simulink model "PTC_EL_PDgJLA_FracPol_20201"  (R2020b)
settings: Solver=VariableStepAuto  StartTime=0.0  StopTime=10.0  RelTol=1e-3
settings Model: Creator=Amir  LastModifiedBy=Amir

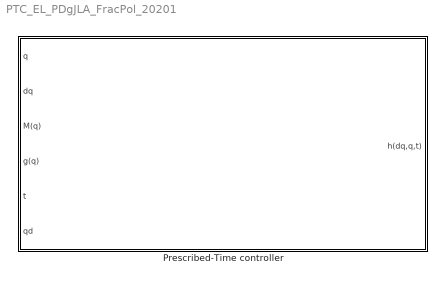
== system PTC_EL_PDgJLA_FracPol_20201 ==
  Prescribed-Time controller : Subsystem  mask(Prescribed-Time Control for Robotics Systems - Version: PTC.EL.PDg-JLA.FracPol.2020-1){n=2, tau=20, P=-0.1*eye(2), D=-1*eye(2), checkBoxA=on, grav_onoff=1, checkBoxB=on, avoid_onoff=1, qmax=[inf;3*pi/180], qmin=[-inf;-3*pi/180], infl=0.5*pi/180, eta=[0;1e-9], a=20, b=1, c=1, epsilon_t=1, epsilon_x=0}
      mask prompts: n "Degrees of Freedom (n):"; tau "Stabilization time (tau):"; P "Proportional (P):"; D "Derivative (D):"; checkBoxA "Gravity compensation"; checkBoxB "Joint limit avoidance"; qmax "Maximum limits (q_max):"; qmin "Minimum limits (q_min):"; infl "Distance limit of influence:"; eta "Joint limit force gain:"
      mask Help:
      | This simulink block obtains a prescribed-time control for Euler-Lagrnage systems of the following form:
      | 
      | M(q)*q+C(dq,q)*dq+g(q)=u+d(t)
      | 
      | where the position of the robot is 'q' and its time derivative is shown by 'dq'. Matrices 'M(q)' and 'C(dq,q)' are the inertia and Coriolis matrices, respectively. Vector 'g(q)' is the gravity force and 'u' stands for the control input. The unmodeled perturbations are refered to by 'd(t)'.
      | 
      | The prescribed-time controller stabilizes the above-mentioned Euler-Lagrange system at 't=tau'.
      | 
      | The parameters of this block are:
      | 
      | 1) n: The degrees of freedom (DOF) of the robot, i.e., the dimension of vector 'q'.
      | 
      | 2) tau: The intended convergence time.
      | 
      | 3) P: The proportional matrix of the infinite-time controller.
      | 
      | 4) D: The derivative matrix of the infinite-time controller.
      | 
      | 5) Gravity compensation checkbox: Infinite-time controller with or whithout gravity compensation.
      | 
      | 6) Joint limit avoidance checkbox: Infinite-time controller with or without joint limit avoidance (use only for revolute joints).
      | 
      | 7) qmax: Maximum limit of the joint angle as a n-dimensional vector.
      | 
      | 8) qmin: Minimum limit of the joint angle as a n-dimensional vector.
      | 
      | 9) Distance limit of influence: Distance limit of the potential field influence; larger values influences the robot even far from the joint limits.
      | 
      | 10) Joint limit force gain: A gain for the joint limit avoidance force.
      | 
      | 11) a: The numinator coefficient for a polynomial mapping function; set an m-dimensional vector to have a mapping function by sum of m polynomial terms.
      | 
      | 12) b: The nominator power for a polynomial mapping function; set an m-dimensional vector to have a mapping function by sum of m polynomial terms.
      | 
      | 13) c: The denominator power for a polynomial mapping function; set an m-dimensional vector to have a mapping function by sum of m polynomial terms.
      | 
      | 14) epsilon_t: For a time-dependent switching, the controller switches to fixed gains at t=tau-epsilon_t.
      | 
      | 15) epsilon_x: For a state-dependent switching, the controller switches to fixed gains when norm(x)<epsilon_x.
      mask Callback checkBoxA:
      | box_A = get_param(gcb, 'checkBoxA');
      | m = Simulink.Mask.get(gcb);
      | 
      | if strcmp(box_A, 'on')
      |     set_param(gcb,'grav_onoff','1')
      | %     grav_onoff=1;
      | else
      |     set_param(gcb,'grav_onoff','0')
      | %     grav_onoff=0;
      | end
      mask Callback checkBoxB:
      | box_B = get_param(gcb, 'checkBoxB');
      | m = Simulink.Mask.get(gcb);
      | m1 = m.getParameter('qmax');
      | m2 = m.getParameter('qmin');
      | m3 = m.getParameter('infl');
      | m4 = m.getParameter('eta');
      | 
      | if strcmp(box_B, 'on')
      |     m1.Enabled = 'on';
      |     m2.Enabled = 'on';
      |     m3.Enabled = 'on';
      |     m4.Enabled = 'on';
      |     set_param(gcb,'avoid_onoff','1')
      | %     avoid_onoff=1;
      | else
      |     m1.Enabled = 'off';
      |     m2.Enabled = 'off';
      |     m3.Enabled = 'off';
      |     m4.Enabled = 'off';
      |     set_param(gcb,'avoid_onoff','0')
      | %     avoid_onoff=0;
      | end
      mask DialogControl DescGroupVar Prompt: Main
      mask DialogControl DescTextVar Prompt: This block obtains a prescribed-time control for robotics system governed by Euler-Lagrange systems.
      mask DialogControl Control5 Prompt: The controller can be set to avoid maximum and minimum limits for revolute joints.
      mask DialogControl Control6 Prompt: The stabilization occurs at 't=tau'. The controller switches to a fixed gain scheme at 't=tau-epsilon_t', or when the norm of state variables reaches a tolerance of 'epsilon_x'.
      mask DialogControl DescTextVar_copy Prompt: This version is based on a Proportional Derivative (PD) controller with/without gravity compensation as the core infinite-time controller. The mapping function is a sum of fractions of polynomials.
      mask DialogControl Container4 Prompt: Parameters
      mask DialogControl ParameterGroupVar Prompt: Basics:
      mask DialogControl ParameterGroupVar_copy_copy Prompt: Joint limits
      mask DialogControl ParameterGroupVar_copy Prompt: Mapping details
      mask DialogControl ParameterGroupVar_copy_copy_copy Prompt: Switching criteria
      mask DialogControl Container6 Prompt: More
      mask DialogControl Control3 Prompt: For updated versions, other versions of prescribed-time control, and more stuff, refer to the following link:
      mask DialogControl Control4 Prompt: https://github.com/a-shakouri
      mask DialogControl Control4 Callback: web https://github.com/a-shakouri
      mask Display:
      | color('red');
      | disp('Joint Limit Avoidance\n Prescribed-Time Control\n for Robotics Systems\n\n Version: PTC.EL.PDg-JLA.FracPol.2020-1')
      | color('blue');
      | port_label('output',1,'controller (u)','texmode','on');
      | port_label('input',1,'position (q)','texmode','on');
      | port_label('input',2,'velocity (dq/dt)','texmode','on');
      | port_label('input',3,'Inertia matrix (M(q))','texmode','on');
      | port_label('input',4,'Gravity (g(q))','texmode','on');
      | port_label('input',5,'Time (t)','texmode','on');
      | port_label('input',6,'Reference position (q_d)','texmode','on');

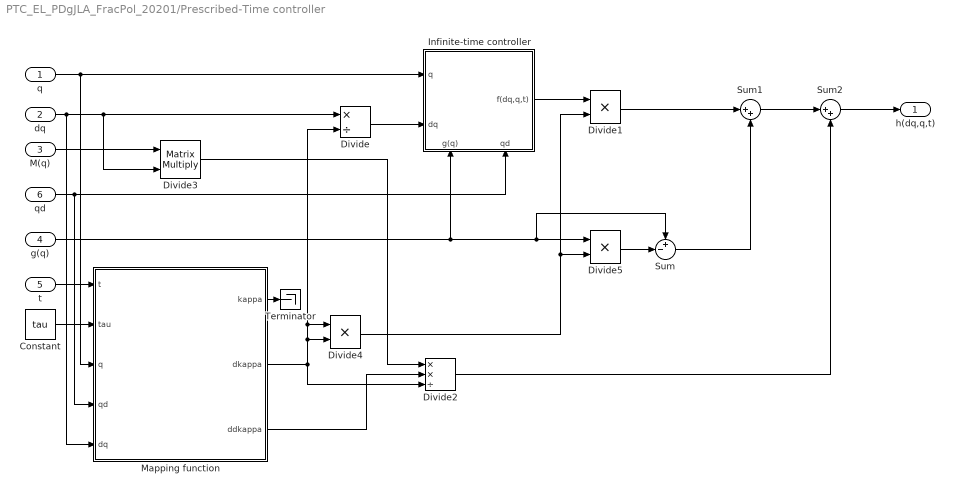
== system PTC_EL_PDgJLA_FracPol_20201/Prescribed-Time controller ==
  q : Inport
  dq : Inport  Port=2
  M(q) : Inport  Port=3
  g(q) : Inport  Port=4
  t : Inport  Port=5
  qd : Inport  Port=6
  Constant : Constant  Value=tau
  Divide : Product  Inputs=*/
  Divide1 : Product  Inputs=**
  Divide2 : Product  Inputs=**/
  Divide3 : Product  Inputs=**  Multiplication=Matrix(*)
  Divide4 : Product  Inputs=**
  Divide5 : Product  Inputs=**
  Infinite-time controller : Subsystem
      settings: PortSchema="{\"entries\":[{\"content\":{\"sides\":[{\"content\":{\"connectorIds\":[\"In1\",\"In2\"]},\"type\":\"ConnectorPlacement.EquallySpacedRectSide\",\"uuid\":\"7fa92645-5ad5-4dcc-b988-cb5fc0cde25c\"},{\"content\":{\"connectorIds\":[\"Out1\"],\"side\":\"RIGHT\"},\"type\":\"ConnectorPlacement.EquallySpacedRectSide\",\"uuid\":\"c20d7c6d-79fc-4692-98a2-c9d8ae7aa432\"},{\"content\":{\"connectorIds\":[],\"side\":\"TOP\"},\"type\":\"ConnectorPlacement.EquallySpacedRectSide\",\"uuid\":\"509ceb5e-78fa-4200-8b36-95fce9268002\"},{\"content\":{\"connectorIds\":[\"In3\",\"In4\"],\"side\":\"BOTTOM\"},\"type\":\"ConnectorPlacement.EquallySpacedRectSide\",\"uuid\":\"0712c4cc-40fb-4aea-b6ca-fbdd2235494d\"},{\"content\":{\"connectorIds\":[],\"side\":\"HIDDEN\"},\"type\":\"ConnectorPlacement.EquallySpacedRectSide\",\"uuid\":\"dedad4c9-c57d-4507-80e4-7406b4950423\"}]},\"type\":\"ConnectorPlacement.EquallySpacedConnector\",\"uuid\":\"14c606af-fbb3-4308-b541-68782b857af4\"}],\"packageUris\":[\"http://schema.mathworks.com/mf0/Connector/R2020b\"],\"version\":\"1.0\"}"
  Mapping function : Subsystem  mask(Polynomial Mapping Function of Class K){a=a, b=b, c=c, Num=0, epsilon_t_copy=epsilon_t, epsilon_x_copy=epsilon_x}
      mask prompts: epsilon_t_copy "epsilon_t:"; epsilon_x_copy "epsilon_x:"
      mask init:
      | Num=length(a);
      mask Help:
      | This simulink block creates the mapping function as well as its first and second derivatives. The mapping functions are of class K such that they go to infinity when the argument approaches t=tau.
      | 
      | The formula of the mapping function (interpreted in LaTeX) is $sum_{i=1}^N(a_i\frac{t^{b_i}}{(\tau-t)^{c_i}})$.
      mask DialogControl DescGroupVar Prompt: Main
      mask DialogControl DescTextVar Prompt: This block obtains the class K mapping function as well as its first and second derivatives for the prescribed-time control of robotics systems. The output limits go to infinity when time approaches 't=tau'. For more details about the following parameters, click on the help button.
      mask DialogControl DescTextVar_copy_copy Prompt: The mapping function ceases updating and returns the latest calculated values after the norm of state variables reaches a tolerance of 'epsilon_x', or the time reaches 't=tau-epsilon_t'.
      mask DialogControl Container12 Prompt: Parameters
      mask DialogControl ParameterGroupVar Prompt: Mapping parameters
      mask DialogControl ParameterGroupVar_copy Prompt: Switching Criteria
      mask DialogControl Container11 Prompt: More
      mask DialogControl DescTextVar_copy Prompt: For updated versions and more stuff refer to the following link:
      mask DialogControl Control3 Prompt: https://github.com/a-shakouri
      mask DialogControl Control3 Callback: web https://github.com/a-shakouri
      mask Display: fprintf('Polynomial class K')
  Sum : Sum  Inputs=+-|
  Sum1 : Sum  Inputs=|++
  Sum2 : Sum  Inputs=|++
  Terminator : Terminator
  h(dq,q,t) : Outport
  wires:
  t/1 -> Mapping function/1(t)
  Constant/1 -> Mapping function/2(tau)
  Divide/1 -> Infinite-time controller/2(dq)
  dq/1 -> Mapping function/5(dq), Divide3/2, Divide/1
  Infinite-time controller/1(f(dq,q,t)) -> Divide1/1
  Mapping function/3(ddkappa) -> Divide2/2
  M(q)/1 -> Divide3/1
  Divide3/1 -> Divide2/1
  Mapping function/1(kappa) -> Terminator/1
  Mapping function/2(dkappa) -> Divide2/3, Divide4/2, Divide4/1, Divide/2
  Divide4/1 -> Divide5/2, Divide1/2
  g(q)/1 -> Sum/1, Divide5/1, Infinite-time controller/3(g(q))
  Divide5/1 -> Sum/2
  Divide1/1 -> Sum1/1
  Sum1/1 -> Sum2/1
  Sum/1 -> Sum1/2
  Divide2/1 -> Sum2/2
  Sum2/1 -> h(dq,q,t)/1
  qd/1 -> Mapping function/4(qd), Infinite-time controller/4(qd)
  q/1 -> Mapping function/3(q), Infinite-time controller/1(q)

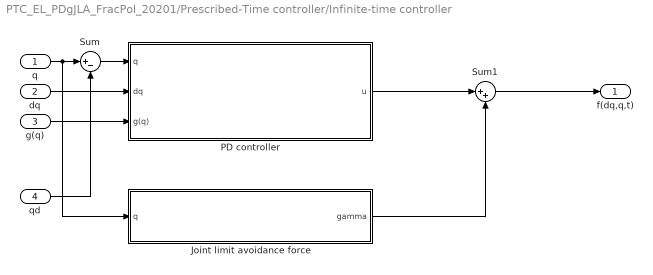
== system PTC_EL_PDgJLA_FracPol_20201/Prescribed-Time controller/Infinite-time controller ==
  q : Inport
  dq : Inport  Port=2
  g(q) : Inport  Port=3
  qd : Inport  Port=4
  Joint limit avoidance force : Subsystem  mask{n=n, qmax=qmax, qmin=qmin, infl=infl, eta=eta}
      mask prompts: n "DOF (n):"; qmax "Maximum limit (q_max):"; qmin "Minimum limit (q_min):"; infl "Distance limit of influence:"; eta "Force gain (eta):"
      mask DialogControl DescGroupVar Prompt: Main
      mask DialogControl DescTextVar Prompt: Joint limit avoidance force for preventing the robot links to violate special angles. This block only works for revolute links. set parameter eta equal to zero for those links that are not revolute or no joint limits are imposed to them.
      mask Display: fprintf('Joint limit avoidance force')
  PD controller : Subsystem  mask{n=n, P=P, D=D, grav_onoff=grav_onoff}
      mask prompts: n "DoF (n):"; P "Proportional gain (P):"; D "Derivative gain (D):"; grav_onoff "Gravity compensation (0 or 1)"
      mask DialogControl DescGroupVar Prompt: Main
      mask DialogControl DescTextVar Prompt: Block of proportional derivative (PD) controller with/without gravity compensation for robotics systems.
      mask Display: fprintf('PD (+Gravity Compensation) Controller')
  Sum : Sum  Inputs=|+-
  Sum1 : Sum  Inputs=|++
  f(dq,q,t) : Outport
  wires:
  dq/1 -> PD controller/2(dq)
  g(q)/1 -> PD controller/3(g(q))
  q/1 -> Joint limit avoidance force/1(q), Sum/1
  Sum/1 -> PD controller/1(q)
  qd/1 -> Sum/2
  PD controller/1(u) -> Sum1/1
  Sum1/1 -> f(dq,q,t)/1
  Joint limit avoidance force/1(gamma) -> Sum1/2

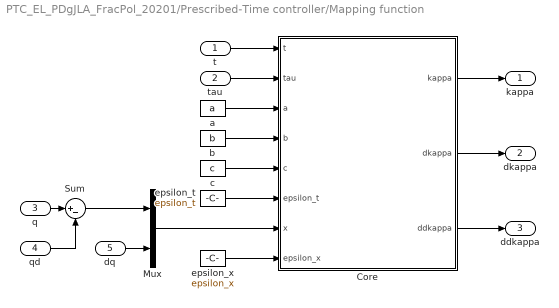
== system PTC_EL_PDgJLA_FracPol_20201/Prescribed-Time controller/Mapping function ==
  t : Inport
  tau : Inport  Port=2
  q : Inport  Port=3
  qd : Inport  Port=4
  dq : Inport  Port=5
  Core : MATLAB Function  TreatAsAtomicUnit=on
  Mux : Mux  Inputs=2
  Sum : Sum  Inputs=|+-
  a : Constant  Value=a
  b : Constant  Value=b
  c : Constant  Value=c
  epsilon_t : Constant  Value=epsilon_t
  epsilon_x : Constant  Value=epsilon_x
  kappa : Outport
  dkappa : Outport  Port=2
  ddkappa : Outport  Port=3
  wires:
  Core/2(dkappa) -> dkappa/1
  Core/1(kappa) -> kappa/1
  Core/3(ddkappa) -> ddkappa/1
  t/1 -> Core/1(t)
  tau/1 -> Core/2(tau)
  a/1 -> Core/3(a)
  b/1 -> Core/4(b)
  c/1 -> Core/5(c)
  epsilon_t/1 -> Core/6(epsilon_t)
  epsilon_x/1 -> Core/8(epsilon_x)
  dq/1 -> Mux/2
  Mux/1 -> Core/7(x)
  q/1 -> Sum/1
  Sum/1 -> Mux/1
  qd/1 -> Sum/2

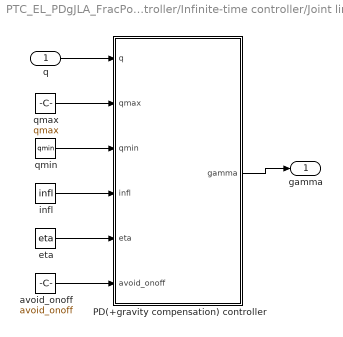
== system PTC_EL_PDgJLA_FracPol_20201/Prescribed-Time controller/Infinite-time controller/Joint limit avoidance force ==
  q : Inport
  PD(+gravity compensation) controller : MATLAB Function  TreatAsAtomicUnit=on
  avoid_onoff : Constant  Value=avoid_onoff
  eta : Constant  Value=eta
  infl : Constant  Value=infl
  qmax : Constant  Value=qmax
  qmin : Constant  Value=qmin
  gamma : Outport
  wires:
  q/1 -> PD(+gravity compensation) controller/1(q)
  infl/1 -> PD(+gravity compensation) controller/4(infl)
  eta/1 -> PD(+gravity compensation) controller/5(eta)
  PD(+gravity compensation) controller/1(gamma) -> gamma/1
  qmin/1 -> PD(+gravity compensation) controller/3(qmin)
  qmax/1 -> PD(+gravity compensation) controller/2(qmax)
  avoid_onoff/1 -> PD(+gravity compensation) controller/6(avoid_onoff)

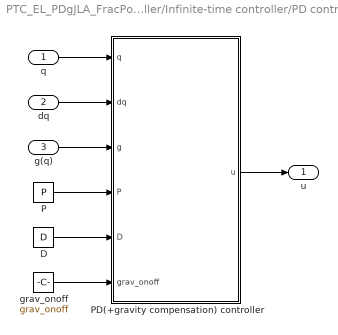
== system PTC_EL_PDgJLA_FracPol_20201/Prescribed-Time controller/Infinite-time controller/PD controller ==
  q : Inport
  dq : Inport  Port=2
  g(q) : Inport  Port=3
  D : Constant  Value=D
  P : Constant  Value=P
  PD(+gravity compensation) controller : MATLAB Function  TreatAsAtomicUnit=on
  grav_onoff : Constant  Value=grav_onoff
  u : Outport
  wires:
  q/1 -> PD(+gravity compensation) controller/1(q)
  P/1 -> PD(+gravity compensation) controller/4(P)
  D/1 -> PD(+gravity compensation) controller/5(D)
  PD(+gravity compensation) controller/1(u) -> u/1
  g(q)/1 -> PD(+gravity compensation) controller/3(g)
  grav_onoff/1 -> PD(+gravity compensation) controller/6(grav_onoff)
  dq/1 -> PD(+gravity compensation) controller/2(dq)

== matlab function PTC_EL_PDgJLA_FracPol_20201/Prescribed-Time controller/Mapping function/Core ==
  data: t input size=[1 1]; kappa output size=[1 1]; dkappa output size=[1 1]; ddkappa output size=[1 1]; tau input size=[1 1]; a input size=[Num 1]; b input size=[Num 1]; c input size=[Num 1]; epsilon_t input; x input; epsilon_x input
function [kappa,dkappa,ddkappa] = mapping_fcn_gen(t,tau,a,b,c,epsilon_t,x,epsilon_x)

if t>tau-epsilon_t || norm(x)<epsilon_x
    
    t=tau-epsilon_t;
    
end
    
kappa=0;
N=length(a);

for i=1:N
    
    kappa=kappa+a(i)*t^b(i)/(tau-t)^c(i);
    
end

dkappa=0;

for i=1:N
    
    dkappa=dkappa+a(i)*((b(i)*t^(b(i)-1))/(tau-t)^c(i)+(c(i)*t^b(i))/(tau-t)^(c(i)+1));
    
end

ddkappa=0;

for i=1:N
    
    if b==1
        
        ddkappa=ddkappa+a(i)*((2*b(i)*c(i)*t^(b(i)-1))/(tau-t)^(c(i)+1)+(c(i)*t^b(i)*(c(i)+1))/(tau-t)^(c(i)+2));
    
    else
        
        ddkappa=ddkappa+a(i)*((b(i)*t^(b(i)-2)*(b(i)-1))/(tau-t)^c(i)+(2*b(i)*c(i)*t^(b(i)-1))/(tau-t)^(c(i)+1)+(c(i)*t^b(i)*(c(i)+1))/(tau-t)^(c(i)+2));
        
    end
    
end

== matlab function PTC_EL_PDgJLA_FracPol_20201/Prescribed-Time controller/Infinite-time controller/PD controller/PD(+gravity compensation) controller ==
  data: q input size=[n 1]; dq input size=[n 1]; g input size=[n 1]; u output size=[n 1]; P input size=[n n]; D input size=[n n]; grav_onoff input size=[1 1]
function u = PD_controller_gen(q,dq,g,P,D,grav_onoff)


u = P*q+D*dq+grav_onoff*g;

== matlab function PTC_EL_PDgJLA_FracPol_20201/Prescribed-Time controller/Infinite-time controller/Joint limit avoidance force/PD(+gravity compensation) controller ==
  data: q input size=[n 1]; qmax input size=[n 1]; qmin input size=[n 1]; gamma output size=[n 1]; infl input size=[1 1]; eta input size=[n 1]; avoid_onoff input
function gamma = PD_controller_gen(q,qmax,qmin,infl,eta,avoid_onoff)


n=length(q);

gamma=zeros(n,1);

if avoid_onoff~=0

for i=1:n
    
    if q(i)<qmin(i)+infl
        
        gamma(i)=eta(i)*(1/(q(i)-qmin(i))-1/(infl))*(1/(q(i)-qmin(i))^2);
        
    elseif q(i)>qmax(i)-infl
        
        gamma(i)=-eta(i)*(1/(qmax(i)-q(i))-1/(infl))*(1/(qmax(i)-q(i))^2);
        
    else
        
        gamma(i)=0;
        
    end
        
end

end
